simulink model "spc4"  (R2020b)
settings: Solver=VariableStepAuto  StartTime=0.0  StopTime=t0  RelTol=1e-3
values from neighbouring files (symbols this model uses):
  i = 21    [SPC_LAB4.m]
  T = [0.001 0.04:0.04:0.8 1]    [SPC_LAB4.m]
  T1 = 11    [SPC_LAB4.m]
  T2 = 5    [SPC_LAB4.m]
  y0 = 1    [SPC_LAB4.m]
settings Model: Creator=Konrad  LastModifiedBy=Konrad

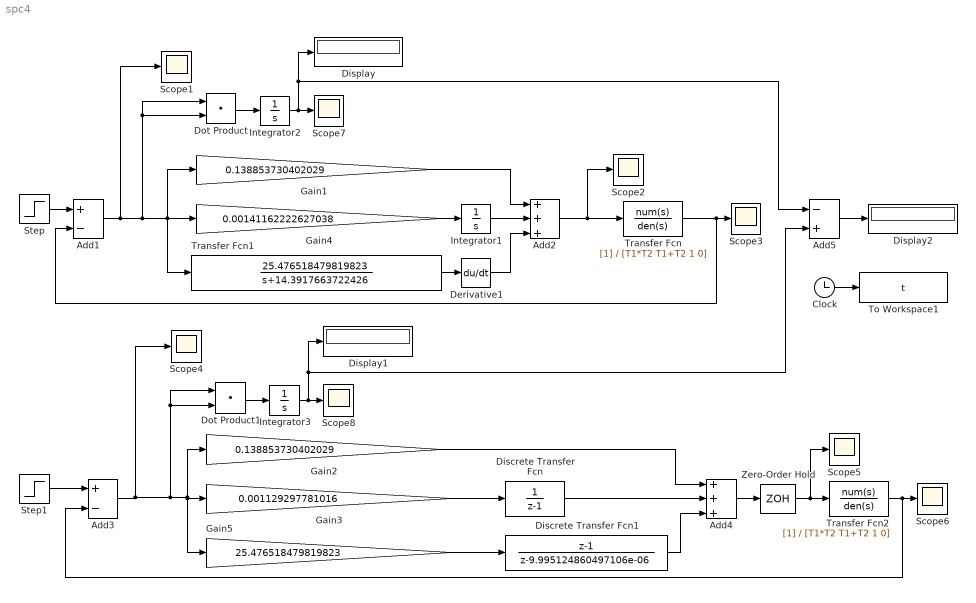
== system spc4 ==
  Add1 : Sum  Inputs=+-
  Add2 : Sum  Inputs=+++
  Add3 : Sum  Inputs=+-
  Add4 : Sum  Inputs=+++
  Add5 : Sum  Inputs=-+
  Clock : Clock
  Derivative1 : Derivative
  Discrete Transfer Fcn : DiscreteTransferFcn  Denominator=[1 -1]  SampleTime=T(i)
  Discrete Transfer Fcn1 : DiscreteTransferFcn  Numerator=[1 -1]  Denominator=[1 -9.995124860497106e-06]  SampleTime=T(i)
  Display : Display
  Display1 : Display
  Display2 : Display
  Dot Product : DotProduct  InputSameDT=on  OutDataTypeStr=Inherit: Inherit via internal rule
  Dot Product1 : DotProduct  InputSameDT=on  OutDataTypeStr=Inherit: Inherit via internal rule
  Gain1 : Gain  Gain=0.138853730402029
  Gain2 : Gain  Gain=0.138853730402029
  Gain3 : Gain  Gain=0.001129297781016
  Gain4 : Gain  Gain=0.00141162222627038
  Gain5 : Gain  Gain=25.476518479819823
  Integrator1 : Integrator
  Integrator2 : Integrator
  Integrator3 : Integrator
  Scope{1..8} (8 alike) : Scope
  Step : Step  After=y0  SampleTime=0
  Step1 : Step  After=y0  SampleTime=0
  To Workspace1 : ToWorkspace  VariableName=t  SaveFormat=Timeseries  SampleTime=-1
  Transfer Fcn : TransferFcn  Denominator=[T1*T2 T1+T2 1 0]
  Transfer Fcn1 : TransferFcn  Numerator=[25.476518479819823]  Denominator=[1 14.3917663722426]
  Transfer Fcn2 : TransferFcn  Denominator=[T1*T2 T1+T2 1 0]
  Zero-Order Hold : ZeroOrderHold  SampleTime=-1
  wires:
  Step/1 -> Add1/1
  Transfer Fcn/1 -> Scope3/1, Add1/2
  Clock/1 -> To Workspace1/1
  Add1/1 -> Dot Product/2, Dot Product/1, Gain1/1, Transfer Fcn1/1, Gain4/1, Scope1/1
  Gain3/1 -> Discrete Transfer Fcn/1
  Gain2/1 -> Add4/1
  Transfer Fcn2/1 -> Scope6/1, Add3/2
  Gain5/1 -> Discrete Transfer Fcn1/1
  Add3/1 -> Gain3/1, Gain5/1, Gain2/1, Dot Product1/2, Dot Product1/1, Scope4/1
  Step1/1 -> Add3/1
  Add4/1 -> Zero-Order Hold/1
  Zero-Order Hold/1 -> Scope5/1, Transfer Fcn2/1
  Discrete Transfer Fcn/1 -> Add4/2
  Discrete Transfer Fcn1/1 -> Add4/3
  Gain1/1 -> Add2/1
  Transfer Fcn1/1 -> Derivative1/1
  Integrator1/1 -> Add2/2
  Gain4/1 -> Integrator1/1
  Derivative1/1 -> Add2/3
  Add2/1 -> Transfer Fcn/1, Scope2/1
  Dot Product/1 -> Integrator2/1
  Dot Product1/1 -> Integrator3/1
  Integrator3/1 -> Display1/1, Add5/2, Scope8/1
  Add5/1 -> Display2/1
  Integrator2/1 -> Display/1, Add5/1, Scope7/1
